simulink model "pendule_inv_capteur_etu"  (R2023b)
settings: Solver=ode45  StartTime=0.0  StopTime=10  RelTol=1e-3
undefined symbols (not defined in the file): g, K, l, ue, x0, xe
settings Model: Creator=fhudrisi  LastModifiedBy=louis
settings OptimizationCC: ReuseModelBlockBuffer=off
settings DebuggingCC: UnconnectedInputMsg=warning  UnconnectedOutputMsg=warning  UnconnectedLineMsg=warning
settings ModelReferenceCC: EnableRefExpFcnMdlSchedulingChecks=on
settings RTWCC: DLArmComputeVersion=19.05

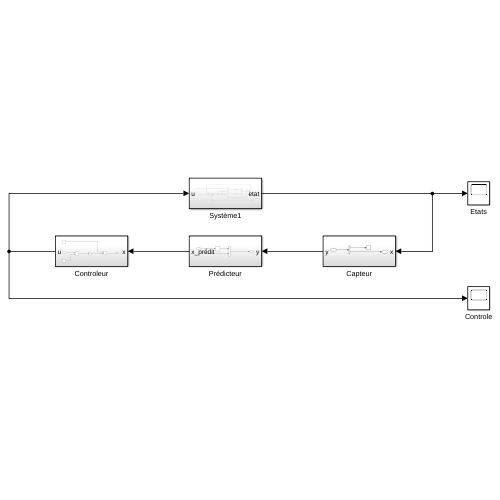
[thumbnail: Simulink's stored preview of the top-level diagram]
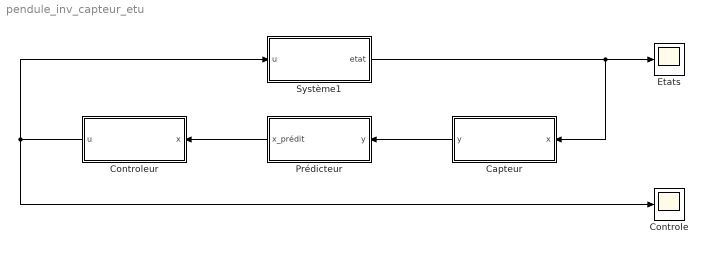
== system pendule_inv_capteur_etu ==
  Capteur : Subsystem
  Controle : Scope
  Controleur : Subsystem
  Etats : Scope
  Prédicteur : Subsystem
  Système1 : Subsystem
  wires:
  Système1/1(etat) -> Etats/1, Capteur/1(x)
  Controleur/1(u) -> Système1/1(u), Controle/1
  Capteur/1(y) -> Prédicteur/1(y)
  Prédicteur/1(x_prédit) -> Controleur/1(x)

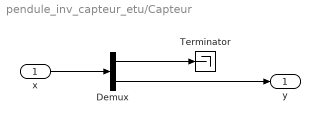
== system pendule_inv_capteur_etu/Capteur ==
  x : Inport
  Demux : Demux  Outputs=2
  Terminator : Terminator
  y : Outport
  wires:
  x/1 -> Demux/1
  Demux/2 -> y/1
  Demux/1 -> Terminator/1

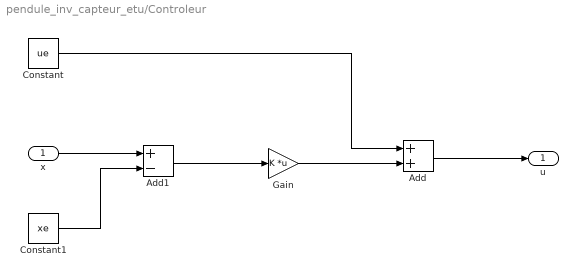
== system pendule_inv_capteur_etu/Controleur ==
  x : Inport
  Add : Sum
  Add1 : Sum  Inputs=+-
  Constant : Constant  Value=ue
  Constant1 : Constant  Value=xe
  Gain : Gain  Gain=K  Multiplication=Matrix(K*u)
  u : Outport
  wires:
  x/1 -> Add1/1
  Constant1/1 -> Add1/2
  Add1/1 -> Gain/1
  Constant/1 -> Add/1
  Gain/1 -> Add/2
  Add/1 -> u/1

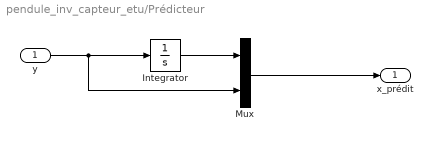
== system pendule_inv_capteur_etu/Prédicteur ==
  y : Inport
  Integrator : Integrator  InitialCondition=x0(1)
  Mux : Mux  Inputs=2
  x_prédit : Outport
  wires:
  y/1 -> Mux/2, Integrator/1
  Integrator/1 -> Mux/1
  Mux/1 -> x_prédit/1

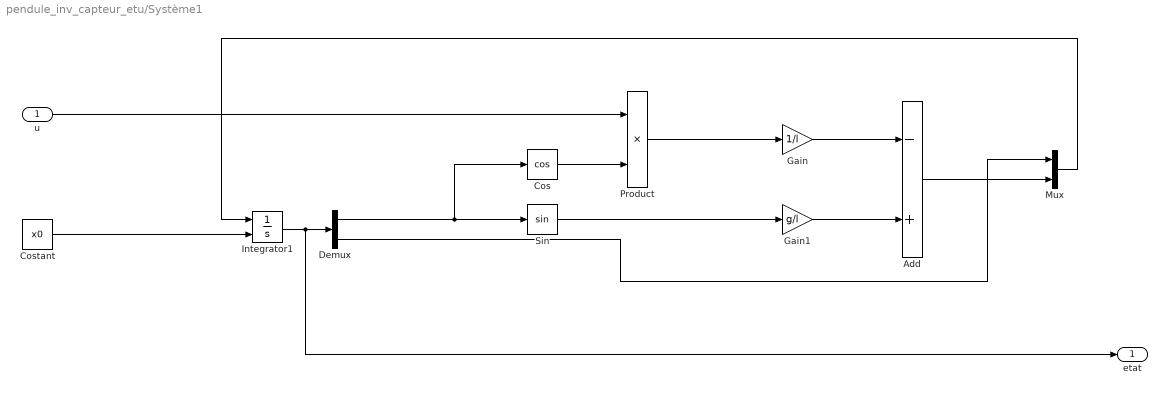
== system pendule_inv_capteur_etu/Système1 ==
  u : Inport
  Add : Sum  Inputs=-+
  Cos : Trigonometry  Operator=cos
  Costant : Constant  Value=x0
  Demux : Demux  Outputs=2
  Gain : Gain  Gain=1/l
  Gain1 : Gain  Gain=g/l
  Integrator1 : Integrator  InitialConditionSource=external
  Mux : Mux  Inputs=2
  Product : Product
  Sin : Trigonometry
  etat : Outport
  wires:
  Costant/1 -> Integrator1/2
  Integrator1/1 -> etat/1, Demux/1
  Demux/1 -> Sin/1, Cos/1
  Cos/1 -> Product/2
  u/1 -> Product/1
  Product/1 -> Gain/1
  Gain/1 -> Add/1
  Sin/1 -> Gain1/1
  Gain1/1 -> Add/2
  Add/1 -> Mux/2
  Demux/2 -> Mux/1
  Mux/1 -> Integrator1/1
